simulink model "MODELO_CORRECTO_BERGMAN_MODIFICADO"  (R2019b)
settings: Solver=VariableStepAuto  StartTime=0.0  StopTime=50000  RelTol=1e-3
undefined symbols (not defined in the file): Gb, Ib, n, p1, p2, p3, Vi
libraries: simulink x6
settings Model: Creator=USUARIO  LastModifiedBy=USUARIO

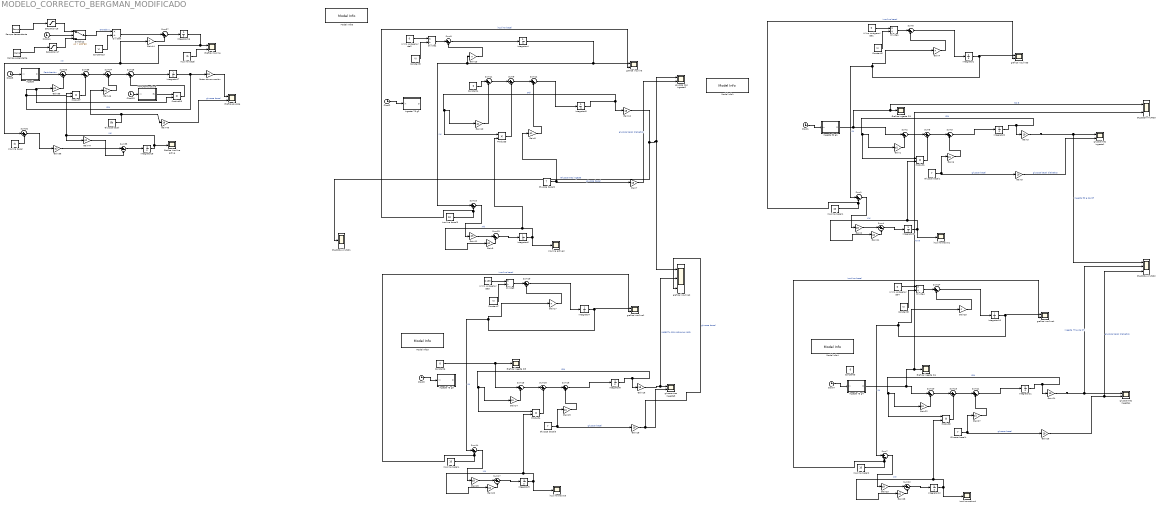
== system MODELO_CORRECTO_BERGMAN_MODIFICADO ==
  Clock{1..5,13,41} (7 alike) : Clock
  Constant{2,5,7..8,13} (5 alike) : Constant  Value=Vi
  Constant3 : Constant  Value=0
  Constant4 : Constant  Value=0
  Constant6 : Constant  Value=0
  Divide{1..4,6} (5 alike) : Product  Inputs=*/
  Factor de conversión : Gain  Gain=18
  GLUCOSA AYUNO1 : Scope  NumInputPorts=3
  GLUCOSA AYUNO2 : Scope  NumInputPorts=3
  GLUCOSA AYUNO3 : Scope  NumInputPorts=2
  Gain{1,6,8,10,14,19,22,27,35,46} (10 alike) : Gain  Gain=p1
  Gain{2,11,15,23,36} (5 alike) : Gain  Gain=p3
  Gain{3,5,7,12,16,18,24,26,45} (9 alike) : Gain  Gain=18
  Gain{4,13,17,25,44} (5 alike) : Gain  Gain=n
  Gain{9,20..21,28,47} (5 alike) : Gain  Gain=p2
  "Glucosa basal  " : Constant  Value=Gb
  Glucosa basal{1..4} (4 alike) : Constant  Value=7
  Grafica ingesta D1 : Scope
  Grafica ingesta D3 : Scope
  Grafica ingesta D4 : Scope
  "Gráfica glucosa " : Scope  NumInputPorts=2
  "Gráfica insulina " : Scope  NumInputPorts=2
  Gráfica insulina activa : Scope
  "Ingesta     " : MATLAB Function  TreatAsAtomicUnit=on
  Ingesta 50 g1 : MATLAB Function  TreatAsAtomicUnit=on
  Ingesta 75 g2 : MATLAB Function  TreatAsAtomicUnit=on
  Ingesta 75 g3 : MATLAB Function  TreatAsAtomicUnit=on
  Ingesta 75 g4 : MATLAB Function  TreatAsAtomicUnit=on
  "Insulina basal    " : Constant  Value=Ib
  "Insulina basal      " : Constant  Value=Ib
  Insulina basal{1..4} (4 alike) : Constant  Value=10
  Integrator{1,4,7,10} (4 alike) : Integrator  InitialCondition=10
  Integrator{2,5,8,11,17} (5 alike) : Integrator  InitialCondition=7
  Integrator{3,6,12,16,18} (5 alike) : Integrator
  Integrator9 : Integrator  InitialCondition=-0.000194
  MATLAB Function5 : MATLAB Function  TreatAsAtomicUnit=on
  Model Info1 : simulink/Model-Wide Utilities/Model Info  Frame=on  DisplayStringWithTags=|  HorizontalTextAlignment=Center  LeftAlignmentValue=0.5
      | MODELO MODIFICADO
      | 
      | INGESTA SIN INSULINA
      | 
      | PERSONA DIABETICA tipo 1
  Model Info3 : simulink/Model-Wide Utilities/Model Info  Frame=on  DisplayStringWithTags=|  HorizontalTextAlignment=Center  LeftAlignmentValue=0.5
      | MODELO MODIFICADO
      | 
      | TRAS INGESTA CON INSULINA
      | 
      | PERSONA DIABETICA
  Model Info4 : simulink/Model-Wide Utilities/Model Info  Frame=on  DisplayStringWithTags=|  HorizontalTextAlignment=Center  LeftAlignmentValue=0.5
      | MODELO MODIFICADO
      | 
      | TRAS INGESTA SIN INSULINA
      | 
      | PERSONA DIABETICA tipo 1
  Model Info6 : simulink/Model-Wide Utilities/Model Info  Frame=on  DisplayStringWithTags=MODELO MODIFICADO  HorizontalTextAlignment=Center  LeftAlignmentValue=0.5
  Product{1..4,7,15} (6 alike) : Product
  "Rampa ascendente    " : simulink/Sources/Ramp  slope=0.000083  start=0  InitialOutput=0
  "Rampa descendente  " : simulink/Sources/Ramp  slope=-0.0000125  start=400*60  InitialOutput=0.3
  Saturation17 : Saturate  UpperLimit=0.3  LowerLimit=0
  Saturation18 : Saturate  UpperLimit=0  LowerLimit=0
  Sum{1..2,4..11,13..15,17..20,22..25,32..33,35..37} (26 alike) : Sum  Inputs=|+-
  Sum{3,12,16,21,34} (5 alike) : Sum  Inputs=|++
  Switch12 : Switch  Criteria=u2 > Threshold  Threshold=400*60
  U (ins. exógena) cte1 : Constant  Value=0
  U (ins. exógena) cte2 : Constant  Value=0
  U (ins. exógena) cte3 : Constant  Value=0.185
  U (ins. exógena) cte4 : Constant  Value=0
  glucosa tras ingesta{1..4} (4 alike) : Scope  NumInputPorts=2
  grafica insulina{,1,3..4} (4 alike) : Scope  NumInputPorts=2
  grafica insulina2 : Scope  NumInputPorts=3
  insulina activa{1..4} (4 alike) : Scope
  wires:
  Sum37/1 -> Integrator16/1
  Integrator18/1 -> Gráfica insulina activa/1, Product7/2, Gain47/1  "X(t)"
  Sum36/1 -> Sum34/1
  "Ingesta     "/1(D) -> Sum33/1  "Perturbación"
  Integrator17/1 -> Factor de conversión/1, Gain35/1, Product15/2, Product7/1  "G(t)"
  Sum35/1 -> Integrator18/1
  "Glucosa basal  "/1 -> Gain46/1, Gain45/1
  Integrator16/1 -> "Gráfica insulina "/1, Sum32/1, Gain44/1  "I(t)"
  Gain45/1 -> "Gráfica glucosa "/2  "glucosa basal"
  Gain44/1 -> Sum37/2
  Gain46/1 -> Sum34/2
  Divide6/1 -> Sum37/1
  Gain35/1 -> Sum33/2
  Sum32/1 -> Gain36/1
  Product7/1 -> Sum36/2
  Gain36/1 -> Sum35/1
  Gain47/1 -> Sum35/2
  Constant13/1 -> Divide6/2
  Sum33/1 -> Sum36/1
  Factor de conversión/1 -> "Gráfica glucosa "/1
  "Insulina basal    "/1 -> Sum32/2
  Gain15/1 -> Sum17/1
  Constant4/1 -> Sum11/1
  Sum9/1 -> Integrator4/1
  Sum19/1 -> Integrator7/1
  Gain8/1 -> Sum12/2
  Integrator7/1 -> grafica insulina1/1, Gain17/1, Sum14/1  "I(t)"
  Sum12/1 -> Integrator5/1
  Gain13/1 -> Sum9/2
  Insulina basal4/1 -> grafica insulina1/2, Sum14/2  "insulina basal"
  Divide2/1 -> Sum9/1
  Integrator6/1 -> insulina activa2/1, Product3/2, Gain9/1  "X(t)"
  Glucosa basal3/1 -> Gain19/1, Gain18/1  "glucosa basal"
  Gain14/1 -> Sum15/2
  Constant6/1 -> Grafica ingesta D3/1, Sum15/1
  Gain19/1 -> Sum16/2
  Product4/1 -> Sum18/2
  Sum11/1 -> Sum8/1
  Sum10/1 -> Gain11/1
  Integrator4/1 -> Sum10/1, Gain13/1, grafica insulina/1  "I(t)"
  Sum16/1 -> Integrator8/1
  Gain11/1 -> Sum13/1
  Sum13/1 -> Integrator6/1
  Gain17/1 -> Sum19/2
  Divide3/1 -> Sum19/1
  Insulina basal3/1 -> grafica insulina/2, Sum10/2  "insulina basal"
  Gain18/1 -> grafica insulina2/3, glucosa tras ingesta3/2  "glucosa basal"
  Sum8/1 -> Sum12/1
  Integrator5/1 -> Gain12/1, Product3/1, Gain10/1  "G(t)"
  Gain20/1 -> Sum17/2
  Integrator8/1 -> Gain16/1, Product4/1, Gain14/1  "G(t)"
  Constant7/1 -> Divide3/2
  Gain10/1 -> Sum11/2
  Clock2/1 -> Ingesta 75 g2/1(in)
  Product3/1 -> Sum8/2
  Sum15/1 -> Sum18/1
  Constant5/1 -> Divide2/2
  U (ins. exógena) cte2/1 -> Divide2/1
  Gain16/1 -> grafica insulina2/2, glucosa tras ingesta3/1  "INGESTA CON INSULINA MOD"
  Sum18/1 -> Sum16/1
  Sum14/1 -> Gain15/1
  Gain7/1 -> glucosa tras ingesta2/2  "glucosa basal diabetico"
  Glucosa basal2/1 -> Gain8/1, Gain7/1  "glucosa basal"
  Sum17/1 -> Integrator9/1
  Gain12/1 -> GLUCOSA AYUNO1/2, grafica insulina2/1, glucosa tras ingesta2/1  "Glucosa tras ingesta"
  U (ins. exógena) cte3/1 -> Divide3/1
  Clock3/1 -> Ingesta 75 g3/1(in)
  Gain9/1 -> Sum13/2
  Integrator9/1 -> insulina activa3/1, Product4/2, Gain20/1  "X(t)"
  Gain21/1 -> Sum4/2
  Integrator1/1 -> grafica insulina3/1, Gain4/1, Sum1/1  "I(t)"
  U (ins. exógena) cte1/1 -> Divide1/1
  Gain3/1 -> GLUCOSA AYUNO2/1, glucosa tras ingesta1/1  "Ingesta 50 g de CH"
  Constant2/1 -> Divide1/2
  Product1/1 -> Sum5/2
  Gain1/1 -> Sum2/2
  Glucosa basal1/1 -> Gain6/1, Gain5/1  "glucosa basal"
  Clock1/1 -> Ingesta 50 g1/1(in)
  Gain5/1 -> glucosa tras ingesta1/2  "glucosa basal diabetico"
  Integrator2/1 -> Gain3/1, Product1/1, Gain1/1  "G(t)"
  Integrator3/1 -> insulina activa1/1, Product1/2, Gain21/1  "X(t)"
  Sum5/1 -> Sum3/1
  Divide1/1 -> Sum6/1
  Gain4/1 -> Sum6/2
  Sum3/1 -> Integrator2/1
  Sum6/1 -> Integrator1/1
  Insulina basal1/1 -> grafica insulina3/2, Sum1/2  "insulina basal"
  Gain2/1 -> Sum4/1
  Gain6/1 -> Sum3/2
  Sum4/1 -> Integrator3/1
  Sum1/1 -> Gain2/1
  Sum2/1 -> Sum5/1
  Gain28/1 -> Sum22/2
  Integrator10/1 -> grafica insulina4/1, Gain25/1, Sum7/1  "I(t)"
  U (ins. exógena) cte4/1 -> Divide4/1
  Gain24/1 -> GLUCOSA AYUNO2/2, glucosa tras ingesta4/1  "Ingesta 75 g de CH"
  Constant8/1 -> Divide4/2
  Product2/1 -> Sum23/2
  Gain22/1 -> Sum20/2
  Glucosa basal4/1 -> Gain27/1, Gain26/1  "glucosa basal"
  Clock4/1 -> Ingesta 75 g4/1(in)
  Gain26/1 -> GLUCOSA AYUNO2/3, glucosa tras ingesta4/2  "glucosa basal diabetico"
  Integrator11/1 -> Gain24/1, Product2/1, Gain22/1  "G(t)"
  Integrator12/1 -> insulina activa4/1, Product2/2, Gain28/1  "X(t)"
  Sum23/1 -> Sum21/1
  Divide4/1 -> Sum24/1
  Gain25/1 -> Sum24/2
  Sum21/1 -> Integrator11/1
  Sum24/1 -> Integrator10/1
  Insulina basal2/1 -> grafica insulina4/2, Sum7/2  "insulina basal"
  Gain23/1 -> Sum22/1
  Gain27/1 -> Sum21/2
  Sum22/1 -> Integrator12/1
  Sum7/1 -> Gain23/1
  Sum20/1 -> Sum23/1
  Ingesta 75 g4/1(D) -> GLUCOSA AYUNO3/2, Grafica ingesta D4/1, Sum20/1  "75 G"
  Ingesta 50 g1/1(D) -> GLUCOSA AYUNO3/1, Grafica ingesta D1/1, Sum2/1  "50 G"
  Clock5/1 -> "Ingesta     "/1(in)
  MATLAB Function5/1(Ej) -> Product15/1
  Clock13/1 -> MATLAB Function5/1(in)
  Sum34/1 -> Sum25/1
  Sum25/1 -> Integrator17/1
  Product15/1 -> Sum25/2
  Clock41/1 -> Switch12/2
  "Rampa ascendente    "/1 -> Saturation17/1
  Saturation18/1 -> Switch12/1
  "Rampa descendente  "/1 -> Saturation18/1
  Switch12/1 -> Divide6/1  "entrada U"
  Saturation17/1 -> Switch12/3
  "Insulina basal      "/1 -> "Gráfica insulina "/2

== matlab function MODELO_CORRECTO_BERGMAN_MODIFICADO/Ingesta 50 g1 ==
  data: in input; D output
function D = comida(in)
% Variables de entrada en la funcion
t = in(1) %- 8*60*60; % Ajuste para iniciar a las 8 de la mañana
 
% Parámetros del modelo
Ag = 0.8; % adimensional
Tmaxi = 55*60; % s
Vg = 13.79; % L
Tmaxg = 40*60; % s
t1 = 0;
Dg = 0;
f = 1000/180; % factor de conversión de g a mmol
 
% Comidas (perturbaciones) a lo largo de un día
if t >= 0 && t < 500*60 % ingesta de 75 g de HC
    t1 = 0;
    Dg = 50*f;
end
 
% Ecuación
D = (Dg*Ag*(t-t1)*exp(-(t-t1)/Tmaxi))/(Vg*Tmaxg^2);

== matlab function MODELO_CORRECTO_BERGMAN_MODIFICADO/Ingesta 75 g2 ==
  data: in input; D output
function D = comida(in)
% Variables de entrada en la funcion
t = in(1) %- 8*60*60; % Ajuste para iniciar a las 8 de la mañana
 
% Parámetros del modelo
Ag = 0.8; % adimensional
Tmaxi = 55*60; % s
Vg = 13.79; % L
Tmaxg = 40*60; % s
t1 = 0;
Dg = 0;
f = 1000/180; % factor de conversión de g a mmol
 
% Comidas (perturbaciones) a lo largo de un día
if t >= 0 && t < 180*60 % ingesta de 75 g de HC
    t1 = 0;
    Dg = 50*f;
end
 
% Ecuación
D = (Dg*Ag*(t-t1)*exp(-(t-t1)/Tmaxi))/(Vg*Tmaxg^2);

== matlab function MODELO_CORRECTO_BERGMAN_MODIFICADO/Ingesta 75 g3 ==
  data: in input; D output
function D = comida(in)
% Variables de entrada en la funcion
t = in(1) %- 8*60*60; % Ajuste para iniciar a las 8 de la mañana
 
% Parámetros del modelo
Ag = 0.8; % adimensional
Tmaxi = 55*60; % s
Vg = 13.79; % L
Tmaxg = 40*60; % s
t1 = 0;
Dg = 0;
f = 1000/180; % factor de conversión de g a mmol
 
% Comidas (perturbaciones) a lo largo de un día
if t >= 0 && t < 180*60 % ingesta de 75 g de HC
    t1 = 0;
    Dg = 50*f;
end
 
% Ecuación
D = (Dg*Ag*(t-t1)*exp(-(t-t1)/Tmaxi))/(Vg*Tmaxg^2);

== matlab function MODELO_CORRECTO_BERGMAN_MODIFICADO/Ingesta 75 g4 ==
  data: in input; D output
function D = comida(in)
% Variables de entrada en la funcion
t = in(1) %- 8*60*60; % Ajuste para iniciar a las 8 de la mañana
 
% Parámetros del modelo
Ag = 0.8; % adimensional
Tmaxi = 55*60; % s
Vg = 13.79; % L
Tmaxg = 40*60; % s
t1 = 0;
Dg = 0;
f = 1000/180; % factor de conversión de g a mmol
 
% Comidas (perturbaciones) a lo largo de un día
if t >= 0 && t < 500*60 % ingesta de 75 g de HC
    t1 = 0;
    Dg = 75*f;
end
 
% Ecuación
D = (Dg*Ag*(t-t1)*exp(-(t-t1)/Tmaxi))/(Vg*Tmaxg^2);

== matlab function MODELO_CORRECTO_BERGMAN_MODIFICADO/Ingesta      ==
  data: in input; D output
function D = comida(in)
% Variables de entrada en la funcion
t = in(1) %- 8*60*60; % Ajuste para iniciar a las 8 de la mañana
 
% Parámetros del modelo
Ag = 0.8; % adimensional
Tmaxi = 55*60; % s
Vg = 13.79; % L
Tmaxg = 40*60; % s
t1 = 0;
Dg = 0;
f = 1000/180; % factor de conversión de g a mmol
 
% Comidas (perturbaciones) a lo largo de un día
if t >= 0 && t < 180*60 % ingesta de 75 g de HC
    t1 = 0;
    Dg = 50*f;
end
 
% Ecuación
D = (Dg*Ag*(t-t1)*exp(-(t-t1)/Tmaxi))/(Vg*Tmaxg^2);

== matlab function MODELO_CORRECTO_BERGMAN_MODIFICADO/MATLAB Function5 ==
  data: in input; Ej output
function Ej  = ejercicio(in)
% Variables de entrada en la funcion
t = in(1);
%Parametros del modelo
cons = 0.005/60;
%Ejercicio (perturbaciones) a lo largo de un día

if t>=0 && t<60*60 %ejercicio 1 h
 Ej=0;
elseif t>=60*60 && t<180*60 %ejercicio 2 h
 Ej=cons+ 0.005/60;
else
 Ej=cons/2;
end
